simulink subsystem "Dissipator_circuit"  (R2020b)
settings: Solver=VariableStepAuto  StartTime=0.0  StopTime=10.0  RelTol=1e-3
settings Model: Creator=avina  LastModifiedBy=avina

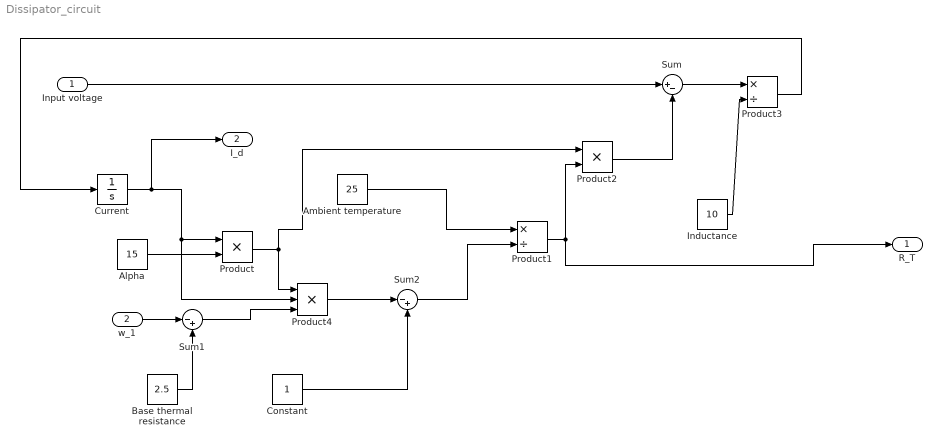
== system Dissipator_circuit ==
  Input voltage : Inport
  w_1 : Inport  Port=2
  Alpha : Constant  Value=15
  Ambient temperature : Constant  Value=25
  Base thermal resistance : Constant  Value=2.5
  Constant : Constant
  Current : Integrator  InitialCondition=1e-7
  Inductance : Constant  Value=10
  Product : Product
  Product1 : Product  Inputs=*/
  Product2 : Product
  Product3 : Product  Inputs=*/
  Product4 : Product  Inputs=3
  Sum : Sum  Inputs=|+-
  Sum1 : Sum  Inputs=|-+
  Sum2 : Sum  Inputs=|-+
  R_T : Outport
  I_d : Outport  Port=2
  wires:
  Alpha/1 -> Product/2
  Base thermal resistance/1 -> Sum1/2
  w_1/1 -> Sum1/1
  Product/1 -> Product2/1, Product4/1
  Ambient temperature/1 -> Product1/1
  Product1/1 -> Product2/2, R_T/1
  Input voltage/1 -> Sum/1
  Product2/1 -> Sum/2
  Sum/1 -> Product3/1
  Inductance/1 -> Product3/2
  Product3/1 -> Current/1
  Current/1 -> I_d/1, Product/1, Product4/2
  Constant/1 -> Sum2/2
  Product4/1 -> Sum2/1
  Sum2/1 -> Product1/2
  Sum1/1 -> Product4/3
